simulink model "addition_model"  (R2024b)
settings: Solver=FixedStepAuto  StartTime=0.0  StopTime=10.0  RelTol=1e-3
undefined symbols (not defined in the file): a1, a2
settings Model: SimulationMode=rapid-accelerator  Creator=z004f2se  LastModifiedBy=z004f2se
settings RTWCC: PackageGeneratedCodeAndArtifacts=on  BuildConfiguration=Faster Runs

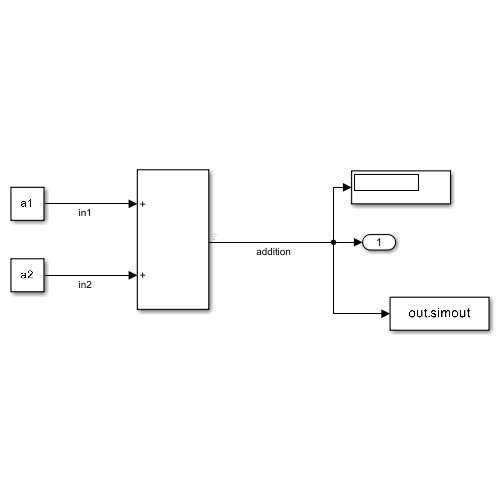
[thumbnail: Simulink's stored preview of the top-level diagram]
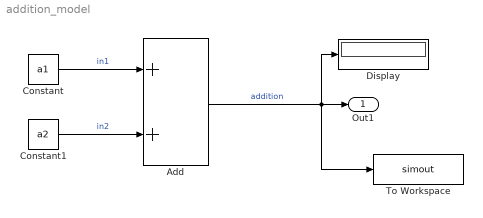
== system addition_model ==
  Add : Sum
  Constant : Constant  Value=a1
  Constant1 : Constant  Value=a2
  Display : Display
  To Workspace : ToWorkspace  VariableName=simout  SaveFormat=Timeseries  SampleTime=-1
  Out1 : Outport
  wires:
  Constant/1 -> Add/1  "in1"
  Constant1/1 -> Add/2  "in2"
  Add/1 -> To Workspace/1, Out1/1, Display/1  "addition"
